simulink model "roll_pitch_pid_control_system"  (R2016b)
settings: Solver=VariableStepAuto  StartTime=0.0  StopTime=10.0  RelTol=1e-3
libraries: simulink x3
settings Model: Creator=E6320  LastModifiedBy=E6320

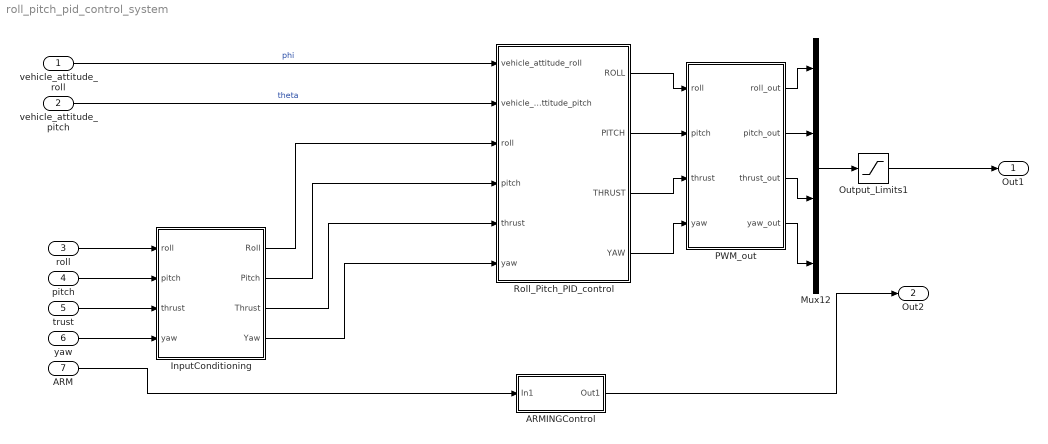
== system roll_pitch_pid_control_system ==
  vehicle_attitude_roll : Inport
  vehicle_attitude_pitch : Inport  Port=2
  roll : Inport  Port=3
  pitch : Inport  Port=4
  trust : Inport  Port=5
  yaw : Inport  Port=6
  ARM : Inport  Port=7
  ARMINGControl : Subsystem
  InputConditioning : Subsystem
  Mux12 : Mux
  Output_Limits1 : Saturate  UpperLimit=2000  LowerLimit=1000
  PWM_out : MATLAB Function  TreatAsAtomicUnit=on
  Roll_Pitch_PID_control : Subsystem
  Out1 : Outport
  Out2 : Outport  Port=2
  wires:
  vehicle_attitude_roll/1 -> Roll_Pitch_PID_control/1(vehicle_attitude_roll)  "phi"
  vehicle_attitude_pitch/1 -> Roll_Pitch_PID_control/2(vehicle_attitude_pitch)  "theta"
  ARM/1 -> ARMINGControl/1(In1)
  roll/1 -> InputConditioning/1(roll)
  pitch/1 -> InputConditioning/2(pitch)
  yaw/1 -> InputConditioning/4(yaw)
  trust/1 -> InputConditioning/3(thrust)
  ARMINGControl/1(Out1) -> Out2/1
  Output_Limits1/1 -> Out1/1
  InputConditioning/1(Roll) -> Roll_Pitch_PID_control/3(roll)
  InputConditioning/2(Pitch) -> Roll_Pitch_PID_control/4(pitch)
  InputConditioning/3(Thrust) -> Roll_Pitch_PID_control/5(thrust)
  InputConditioning/4(Yaw) -> Roll_Pitch_PID_control/6(yaw)
  Roll_Pitch_PID_control/4(YAW) -> PWM_out/4(yaw)
  Roll_Pitch_PID_control/3(THRUST) -> PWM_out/3(thrust)
  Roll_Pitch_PID_control/2(PITCH) -> PWM_out/2(pitch)
  Roll_Pitch_PID_control/1(ROLL) -> PWM_out/1(roll)
  PWM_out/1(roll_out) -> Mux12/1
  PWM_out/2(pitch_out) -> Mux12/2
  PWM_out/3(thrust_out) -> Mux12/3
  PWM_out/4(yaw_out) -> Mux12/4
  Mux12/1 -> Output_Limits1/1

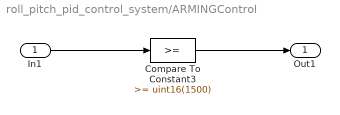
== system roll_pitch_pid_control_system/ARMINGControl ==
  In1 : Inport
  Compare To Constant3 : simulink/Logic and Bit Operations/Compare To Constant  relop=>=  const=uint16(1500)  OutDataTypeStr=boolean
  Out1 : Outport
  wires:
  Compare To Constant3/1 -> Out1/1
  In1/1 -> Compare To Constant3/1

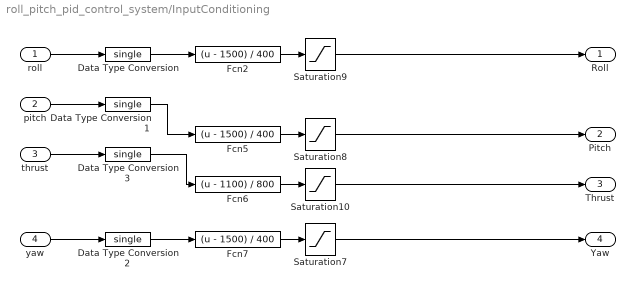
== system roll_pitch_pid_control_system/InputConditioning ==
  roll : Inport
  pitch : Inport  Port=2
  thrust : Inport  Port=3
  yaw : Inport  Port=4
  Data Type Conversion{,1..3} (4 alike) : DataTypeConversion  OutDataTypeStr=single
  Fcn2 : Fcn  Expr=(u - 1500) / 400
  Fcn5 : Fcn  Expr=(u - 1500) / 400
  Fcn6 : Fcn  Expr=(u - 1100) / 800
  Fcn7 : Fcn  Expr=(u - 1500) / 400
  Saturation10 : Saturate  UpperLimit=1  LowerLimit=0
  Saturation7 : Saturate  UpperLimit=1  LowerLimit=-1
  Saturation8 : Saturate  UpperLimit=1  LowerLimit=-1
  Saturation9 : Saturate  UpperLimit=1  LowerLimit=-1
  Roll : Outport
  Pitch : Outport  Port=2
  Thrust : Outport  Port=3
  Yaw : Outport  Port=4
  wires:
  Saturation10/1 -> Thrust/1
  Saturation7/1 -> Yaw/1
  Saturation8/1 -> Pitch/1
  Fcn6/1 -> Saturation10/1
  thrust/1 -> Data Type Conversion3/1
  Fcn2/1 -> Saturation9/1
  Fcn5/1 -> Saturation8/1
  Saturation9/1 -> Roll/1
  Fcn7/1 -> Saturation7/1
  yaw/1 -> Data Type Conversion2/1
  pitch/1 -> Data Type Conversion1/1
  roll/1 -> Data Type Conversion/1
  Data Type Conversion/1 -> Fcn2/1
  Data Type Conversion1/1 -> Fcn5/1
  Data Type Conversion2/1 -> Fcn7/1
  Data Type Conversion3/1 -> Fcn6/1

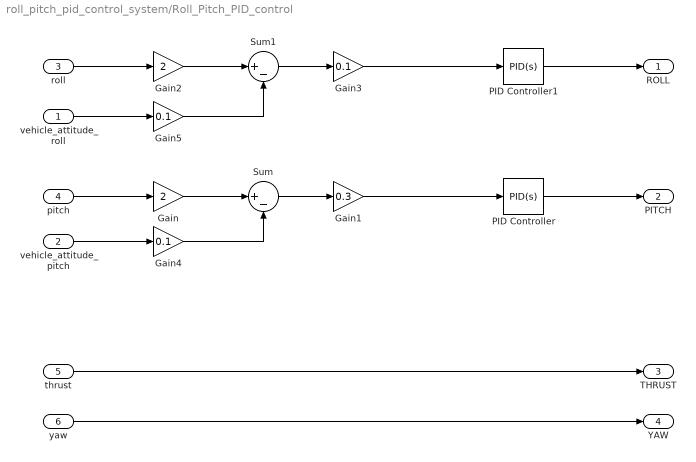
== system roll_pitch_pid_control_system/Roll_Pitch_PID_control ==
  vehicle_attitude_roll : Inport
  vehicle_attitude_pitch : Inport  Port=2
  roll : Inport  Port=3
  pitch : Inport  Port=4
  thrust : Inport  Port=5
  yaw : Inport  Port=6
  Gain : Gain  Gain=2
  Gain1 : Gain  Gain=0.3
  Gain2 : Gain  Gain=2
  Gain3 : Gain  Gain=0.1
  Gain4 : Gain  Gain=0.1
  Gain5 : Gain  Gain=0.1
  PID Controller : simulink/Continuous/PID Controller  Controller=PID  TimeDomain=Continuous-time  SampleTime=-1  IntegratorMethod=Forward Euler  FilterMethod=Forward Euler  Form=Parallel  UseFilter=on  ControllerParametersSource=internal  P=0.8  I=1  D=0.7  N=100  InitialConditionSource=internal  InitialConditionForIntegrator=0  InitialConditionForFilter=0  ExternalReset=none  LimitOutput=off  UpperSaturationLimit=inf  LowerSaturationLimit=-inf  LinearizeAsGain=on  AntiWindupMode=none  Kb=1  TrackingMode=off  Kt=1  PParamMin=[]  PParamMax=[]  IParamMin=[]  IParamMax=[]  DParamMin=[]  DParamMax=[]  NParamMin=[]  NParamMax=[]  KbParamMin=[]  KbParamMax=[]  KtParamMin=[]  KtParamMax=[]  POutMin=[]  POutMax=[]  IOutMin=[]  IOutMax=[]  DOutMin=[]  DOutMax=[]  NOutMin=[]  NOutMax=[]  KbOutMin=[]  KbOutMax=[]  KtOutMin=[]  KtOutMax=[]  IntegratorOutMin=[]  IntegratorOutMax=[]  FilterOutMin=[]  FilterOutMax=[]  SumOutMin=[]  SumOutMax=[]  SumI1OutMin=[]  SumI1OutMax=[]  SumI2OutMin=[]  SumI2OutMax=[]  SumI3OutMin=[]  SumI3OutMax=[]  SumDOutMin=[]  SumDOutMax=[]  SaturationOutMin=[]  SaturationOutMax=[]  IntegratorContinuousStateAttributes=''  IntegratorStateMustResolveToSignalObject=off  IntegratorRTWStateStorageClass=Auto  FilterContinuousStateAttributes=''  FilterStateMustResolveToSignalObject=off  FilterRTWStateStorageClass=Auto  DifferentiatorICPrevScaledInput=0  DifferentiatorOutMin=[]  DifferentiatorOutMax=[]
  PID Controller1 : simulink/Continuous/PID Controller  Controller=PID  TimeDomain=Continuous-time  SampleTime=-1  IntegratorMethod=Forward Euler  FilterMethod=Forward Euler  Form=Parallel  UseFilter=on  ControllerParametersSource=internal  P=0.8  I=1  D=0.7  N=100  InitialConditionSource=internal  InitialConditionForIntegrator=0  InitialConditionForFilter=0  ExternalReset=none  LimitOutput=off  UpperSaturationLimit=inf  LowerSaturationLimit=-inf  LinearizeAsGain=on  AntiWindupMode=none  Kb=1  TrackingMode=off  Kt=1  PParamMin=[]  PParamMax=[]  IParamMin=[]  IParamMax=[]  DParamMin=[]  DParamMax=[]  NParamMin=[]  NParamMax=[]  KbParamMin=[]  KbParamMax=[]  KtParamMin=[]  KtParamMax=[]  POutMin=[]  POutMax=[]  IOutMin=[]  IOutMax=[]  DOutMin=[]  DOutMax=[]  NOutMin=[]  NOutMax=[]  KbOutMin=[]  KbOutMax=[]  KtOutMin=[]  KtOutMax=[]  IntegratorOutMin=[]  IntegratorOutMax=[]  FilterOutMin=[]  FilterOutMax=[]  SumOutMin=[]  SumOutMax=[]  SumI1OutMin=[]  SumI1OutMax=[]  SumI2OutMin=[]  SumI2OutMax=[]  SumI3OutMin=[]  SumI3OutMax=[]  SumDOutMin=[]  SumDOutMax=[]  SaturationOutMin=[]  SaturationOutMax=[]  IntegratorContinuousStateAttributes=''  IntegratorStateMustResolveToSignalObject=off  IntegratorRTWStateStorageClass=Auto  FilterContinuousStateAttributes=''  FilterStateMustResolveToSignalObject=off  FilterRTWStateStorageClass=Auto  DifferentiatorICPrevScaledInput=0  DifferentiatorOutMin=[]  DifferentiatorOutMax=[]
  Sum : Sum  Inputs=|+-
  Sum1 : Sum  Inputs=|+-
  ROLL : Outport
  PITCH : Outport  Port=2
  THRUST : Outport  Port=3
  YAW : Outport  Port=4
  wires:
  pitch/1 -> Gain/1
  Gain/1 -> Sum/1
  vehicle_attitude_pitch/1 -> Gain4/1
  Sum/1 -> Gain1/1
  Gain1/1 -> PID Controller/1
  roll/1 -> Gain2/1
  Gain2/1 -> Sum1/1
  Sum1/1 -> Gain3/1
  Gain4/1 -> Sum/2
  vehicle_attitude_roll/1 -> Gain5/1
  Gain5/1 -> Sum1/2
  Gain3/1 -> PID Controller1/1
  PID Controller1/1 -> ROLL/1
  PID Controller/1 -> PITCH/1
  thrust/1 -> THRUST/1
  yaw/1 -> YAW/1

== matlab function roll_pitch_pid_control_system/PWM_out ==
  data: roll input; roll_out output; pitch input; thrust input; yaw input; pitch_out output; thrust_out output; yaw_out output
function [roll_out,pitch_out,thrust_out,yaw_out] = fcn(roll,pitch,thrust,yaw)
roll_out=uint16(1500+(roll)*400);
pitch_out=uint16(1500+(pitch)*400);
thrust_out=uint16(1100+(thrust)*800);
yaw=uint16(1500+(thrust)*400);
